simulink library "carma_platform"  (Simulink 8.2)
settings: Solver=ode1  StartTime=0.0  StopTime=Inf  FixedStep=0.001  RelTol=1e-3
PostLoadFcn:
  | , if any(exist('dsrtsu_mdlpostloadfcn', 'file') == [2, 3, 6]), try dsrtsu_mdlpostloadfcn('Execute', bdroot); catch fprintf('Error in PostLoadFcn (dsrtsu_mdlpostloadfcn) for model "%s":\n %s\n', bdroot, lasterr); end, end,
libraries: srx_platform x7, topr5_adapter x4, rtitttasklib x4, dsrc_handler x1, parse_utils x1, rtiethernetudplib x1
settings Model: DSRTSU_INTERNAL_RTI_VER=450  DSRTSU_INTERNAL_RTI_TYPE=rti1401  DSRTSU_INTERNAL_RTIFPGA=40  Creator=leidos  LastModifiedBy=rushk1

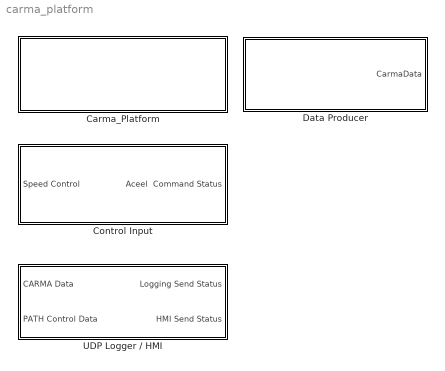
== system carma_platform ==
  "Carma_Platform " : Subsystem
  Control Input : Subsystem
  Data Producer : Subsystem  mask{Value=0.05}
      mask prompts: Value "Data Output Interval (s):"
      mask TypeOptions Value:
      | Triggered
      | Subsystem/Constant2/Value
  UDP Logger / HMI : Subsystem  mask{Value=0.05}
      mask prompts: Value "Output Interval (s):"
      mask TypeOptions Value: Subsystem/Constant2/Value

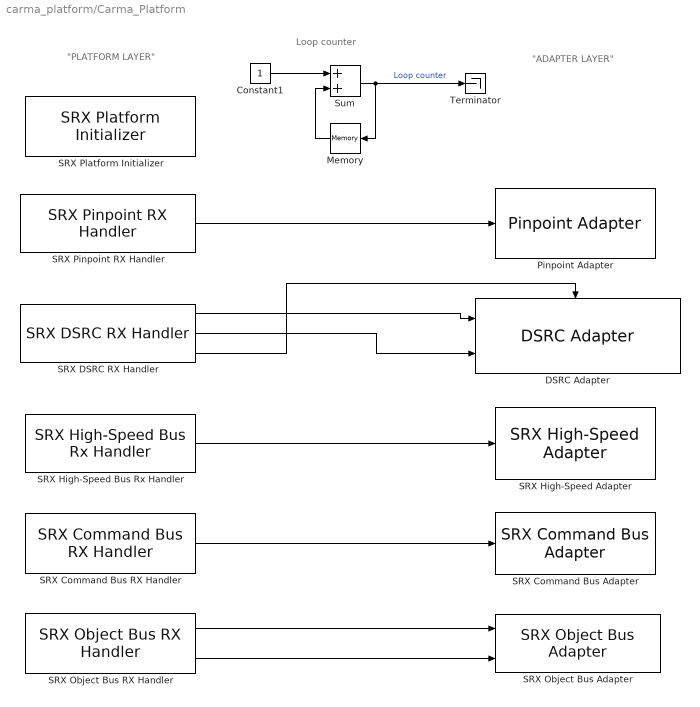
== system carma_platform/Carma_Platform  ==
  note: "ADAPTER LAYER"
  note: "PLATFORM LAYER"
  note: Loop counter
  Constant1 : Constant
  DSRC Adapter : dsrc_handler/DSRC Adapter
  Memory : Memory  InheritSampleTime=on
  Pinpoint Adapter : topr5_adapter/Pinpoint Adapter
  SRX Command Bus Adapter : topr5_adapter/SRX Command Bus Adapter
  SRX Command Bus RX Handler : srx_platform/SRX Command Bus RX Handler  SystemSampleTime=-1
  SRX DSRC RX Handler : srx_platform/SRX DSRC RX Handler
  SRX High-Speed Adapter : topr5_adapter/SRX High-Speed Adapter
  SRX High-Speed Bus Rx Handler : srx_platform/SRX High-Speed Bus Rx Handler  SystemSampleTime=-1
  SRX Object Bus Adapter : topr5_adapter/SRX Object Bus Adapter
  SRX Object Bus RX Handler : srx_platform/SRX Object Bus RX Handler
  SRX Pinpoint RX Handler : srx_platform/SRX Pinpoint RX Handler
  SRX Platform Initializer : srx_platform/SRX Platform Initializer  enable_can1=on  enable_can2=on  enable_can3=on  enable_can4=off
  Sum : Sum  SaturateOnIntegerOverflow=on  InputSameDT=on  OutDataTypeStr=Inherit: Same as first input
  Terminator : Terminator
  wires:
  SRX Pinpoint RX Handler/1 -> Pinpoint Adapter/1
  Sum/1 -> Terminator/1, Memory/1  "Loop counter"
  Memory/1 -> Sum/2
  Constant1/1 -> Sum/1
  SRX High-Speed Bus Rx Handler/1 -> SRX High-Speed Adapter/1
  SRX Command Bus RX Handler/1 -> SRX Command Bus Adapter/1
  SRX Object Bus RX Handler/1 -> SRX Object Bus Adapter/1
  SRX Object Bus RX Handler/2 -> SRX Object Bus Adapter/2
  SRX DSRC RX Handler/1 -> DSRC Adapter/1
  SRX DSRC RX Handler/2 -> DSRC Adapter/2
  SRX DSRC RX Handler/3 -> DSRC Adapter/Enable

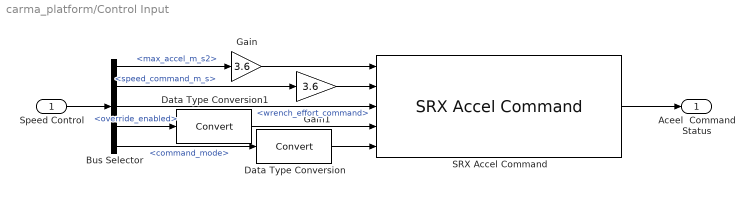
== system carma_platform/Control Input ==
  Speed Control : Inport  OutDataTypeStr=Bus: AccelCommandBus
  Bus Selector : BusSelector  OutputSignals=max_accel_m_s2,speed_command_m_s,wrench_effort_command,override_enabled,command_mode
  Data Type Conversion : DataTypeConversion
  Data Type Conversion1 : DataTypeConversion
  Gain : Gain  Gain=3.6
  Gain1 : Gain  Gain=3.6
  SRX Accel Command : srx_platform/SRX Accel Command
  Aceel  Command Status : Outport
  wires:
  SRX Accel Command/1 -> Aceel  Command Status/1
  Speed Control/1 -> Bus Selector/1
  Gain/1 -> SRX Accel Command/1
  Gain1/1 -> SRX Accel Command/2
  Bus Selector/1 -> Gain/1  "<max_accel_m_s2>"
  Bus Selector/2 -> Gain1/1  "<speed_command_m_s>"
  Bus Selector/3 -> SRX Accel Command/3  "<wrench_effort_command>"
  Bus Selector/4 -> Data Type Conversion1/1  "<override_enabled>"
  Bus Selector/5 -> Data Type Conversion/1  "<command_mode>"
  Data Type Conversion/1 -> SRX Accel Command/5
  Data Type Conversion1/1 -> SRX Accel Command/4

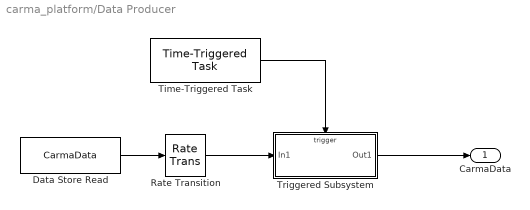
== system carma_platform/Data Producer ==
  Data Store Read : DataStoreRead  DataStoreName=CarmaData  SampleTime=0.01  DataStoreElements=CarmaData
  Rate Transition : RateTransition  Deterministic=off
  Time-Triggered Task : rtitttasklib/Time-Triggered Task  TimeTriggerId=data_prod  TLCFileName=rtitimetriggeredtask  DSProperties=struct('RTI',struct('Version',uint32(1),'BlockType',struct('isSLSource',uint8(1),'isSLSink',uint8(0),'isHWSource',uint8(0),'isHWSink',uint8(0),'isSetup',uint8(0),'isInline',uint8(1),'isNonInline',uint8(0),'isInterrupt',uint8(0),'isChannelwise',uint8(0)),'IOBoardType','RTITIMETRIGGER','UnitType','TIMETRIGGERED','Identifier','TASK','DialogType','SL','BlockSet','NONE','SlaveProcessor','NONE'))  RTIBlockInterface=struct('OutputPortsActive',1,'OutputPortsWidth',int32(1),'FunctionCall',uint32(0),'OutputPortsName',{{[' ']}},'InitLevel',3,'BlockDisplay',{{['Time-Triggered Task\nID: ''''data_prod'''''],'center'}},'IconTransparency','off','BlockName',struct('Token',{{['Time-Triggered Task']}}),'MaskDescription',['Specifies a time-triggered task. The task trigger times are set by the assigned Time-Trigger Set block.' char(10) '' char(10) 'This block can only be used together with the Time-Trigger Set block.'])  RTIBlockParameters=struct('TimeTriggerId',{{'data_prod','OFF',[]}},'TLCFileName',{{'rtitimetriggeredtask','OFF',[]}})  RTISFcnParameters=struct('TLCFileName','char')  RTIBlockParaDefault=struct('TimeTriggerId','TT_ID','TLCFileName','rtitimetriggeredtask')
  Triggered Subsystem : Subsystem  TreatAsAtomicUnit=on
  CarmaData : Outport
  wires:
  Rate Transition/1 -> Triggered Subsystem/1(In1)
  Data Store Read/1 -> Rate Transition/1
  Triggered Subsystem/1(Out1) -> CarmaData/1
  Time-Triggered Task/1 -> Triggered Subsystem/Trigger

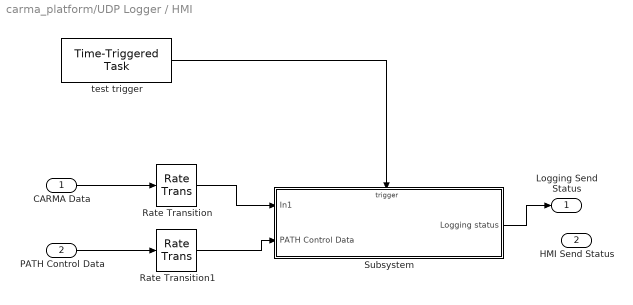
== system carma_platform/UDP Logger / HMI ==
  CARMA Data : Inport
  PATH Control Data : Inport  Port=2  PortDimensions=[74]
  Rate Transition : RateTransition  Deterministic=off
  Rate Transition1 : RateTransition  Deterministic=off
  Subsystem : Subsystem
  test trigger : rtitttasklib/Time-Triggered Task  TimeTriggerId=TT_ID  TLCFileName=rtitimetriggeredtask  DSProperties=struct('RTI',struct('Version',uint32(1),'BlockType',struct('isSLSource',uint8(1),'isSLSink',uint8(0),'isHWSource',uint8(0),'isHWSink',uint8(0),'isSetup',uint8(0),'isInline',uint8(1),'isNonInline',uint8(0),'isInterrupt',uint8(0),'isChannelwise',uint8(0)),'IOBoardType','RTITIMETRIGGER','UnitType','TIMETRIGGERED','Identifier','TASK','DialogType','SL','BlockSet','NONE','SlaveProcessor','NONE'))  RTIBlockInterface=struct('OutputPortsActive',1,'OutputPortsWidth',int32(1),'FunctionCall',uint32(0),'OutputPortsName',{{[' ']}},'InitLevel',3,'BlockDisplay',{{['Time-Triggered Task\nID: ''''TT_ID'''''],'center'}},'IconTransparency','off','BlockName',struct('Token',{{['Time-Triggered Task']}}),'MaskDescription',['Specifies a time-triggered task. The task trigger times are set by the assigned Time-Trigger Set block.' char(10) '' char(10) 'This block can only be used together with the Time-Trigger Set block.'])  RTIBlockParameters=struct('TimeTriggerId',{{'TT_ID','OFF',[]}},'TLCFileName',{{'rtitimetriggeredtask','OFF',[]}})  RTISFcnParameters=struct('TLCFileName','char')  RTIBlockParaDefault=struct('TimeTriggerId','TT_ID','TLCFileName','rtitimetriggeredtask')
  Logging Send Status : Outport
  HMI Send Status : Outport  Port=2
  wires:
  CARMA Data/1 -> Rate Transition/1
  Rate Transition/1 -> Subsystem/1(In1)
  test trigger/1 -> Subsystem/Trigger
  Rate Transition1/1 -> Subsystem/2(PATH Control Data)
  PATH Control Data/1 -> Rate Transition1/1
  Subsystem/1(Logging status) -> Logging Send Status/1
  ? -> HMI Send Status/1

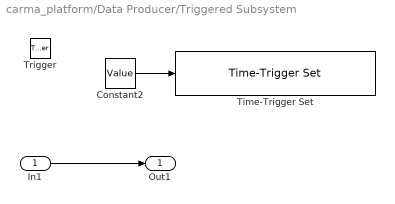
== system carma_platform/Data Producer/Triggered Subsystem ==
  In1 : Inport
  Trigger : TriggerPort  TriggerType=function-call
  Constant2 : Constant  Value=Value
  Time-Trigger Set : rtitttasklib/Time-Trigger Set  TimeTriggerId=data_prod  SampleTime=-1  RegisterAtSimulationStart=on  TLCFileName=rtitimetriggerset  DSProperties=struct('RTI',struct('Version',uint32(1),'BlockType',struct('isSLSource',uint8(1),'isSLSink',uint8(0),'isHWSource',uint8(0),'isHWSink',uint8(0),'isSetup',uint8(0),'isInline',uint8(1),'isNonInline',uint8(0),'isInterrupt',uint8(0),'isChannelwise',uint8(0)),'IOBoardType','RTITIMETRIGGER','UnitType','TIMETRIGGERED','Identifier','SET','DialogType','SL','BlockSet','NONE','SlaveProcessor','NONE'))  RTIBlockInterface=struct('InputPortsActive',1,'InputPortsWidth',{{'DYNAMICALLY_SIZED'}},'InputPortsDataType',{{'SS_DOUBLE'}},'InputPortsName',{{['Trigger delay']}},'InitLevel',3,'BlockDisplay',{{['Time-Trigger Set\nID: ''''data_prod'''''],'center'}},'IconTransparency','on','BlockName',struct('Token',{{['Time-Trigger Set']}}),'MaskDescription',['When this block is evaluated it sets the task trigger times for the assigned time-triggered task.' char(10) '' char(10) 'This block can only be used together with the Time-Triggered Task block.'],'SampleTime',{{-1}})  RTIBlockParameters=struct('TimeTriggerId',{{'data_prod','OFF',[]}},'SampleTime',{{-1,'OFF',[]}},'RegisterAtSimulationStart',{{logical(1),'OFF',[]}},'TLCFileName',{{'rtitimetriggerset','OFF',[]}})  RTISFcnParameters=struct('TimeTriggerId','char','SampleTime','double','TLCFileName','char','RegisterAtSimulationStart','double')  RTIBlockParaDefault=struct('TimeTriggerId','TT_ID','SampleTime',-1,'RegisterAtSimulationStart',0,'TLCFileName','rtitimetriggerset')
  Out1 : Outport
  wires:
  In1/1 -> Out1/1
  Constant2/1 -> Time-Trigger Set/1

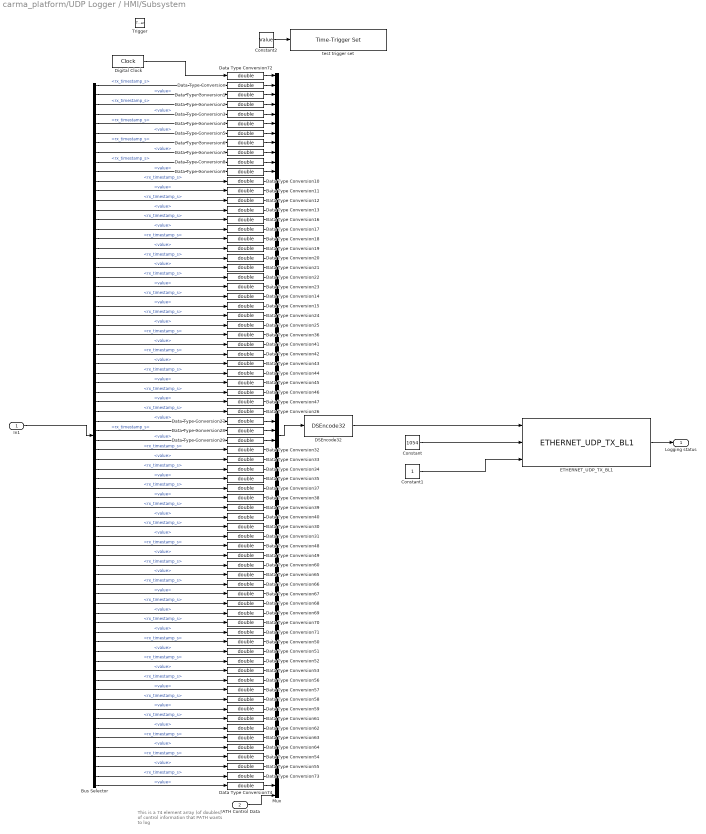
== system carma_platform/UDP Logger / HMI/Subsystem ==
  note: This is a 74 element array (of doubles)
      | of control information that
      | PATH wants to log
  In1 : Inport
  PATH Control Data : Inport  Port=2  PortDimensions=[74]
  Trigger : TriggerPort  TriggerType=function-call  PortDimensions=1
  Bus Selector : BusSelector  OutputSignals=radar_status.rx_timestamp_s,radar_status.value,acc_status.rx_timestamp_s,acc_status.value,path_ctrl_status.rx_timestamp_s,path_ctrl_status.value,throttle_ovr_flag.rx_timestamp_s,throttle_ovr_flag.value,acc_set_speed_m_s.rx_timestamp_s,acc_set_speed_m_s.value,accel_m_s2.rx_timestamp_s,accel_m_s2.value,speed_m_s.rx_timestamp_s,speed_m_s.value,steering_wheel_angle_deg.rx_timestamp_s,steering_wheel_angle_deg.value,brk_light_flag.rx_timestamp_s,brk_light_flag.value,brk_pedal_deflect_percent.rx_timestamp_s,brk_pedal_deflect_percent.value,throttle_pedal_deflect_percent.rx_timestamp_s,throttle_pedal_deflect_percent.value,global_utc_time_s.rx_timestamp_s,global_utc_time_s.value,global_lat_deg.rx_timestamp_s,global_lat_deg.value,global_long_deg.rx_timestamp_s,global_long_deg.value,global_alt_m.rx_timestamp_s,global_alt_m.value,global_roll_deg.rx_timestamp_s,global_roll_deg.value,global_pitch_deg.rx_timestamp_s,global_pitch_deg.value,global_yaw_deg.rx_timestamp_s,global_yaw_deg.value,local_north_m.rx_timestamp_s,local_north_m.value,local_east_m.rx_timestamp_s,local_east_m.value,local_down_m.rx_timestamp_s,local_down_m.value,local_roll_deg.rx_timestamp_s,local_roll_deg.value,local_pitch_deg.rx_timestamp_s,local_pitch_deg.value,local_yaw_deg.rx_timestamp_s,local_yaw_deg.value,horizontal_pos_accuracy_m.rx_timestamp_s,horizontal_pos_accuracy_m.value,vertical_pos_accuracy_m.rx_timestamp_s,vertical_pos_accuracy_m.value,velocity_fwd_m_s.rx_timestamp_s,velocity_fwd_m_s.value,velocity_right_m_s.rx_timestamp_s,velocity_right_m_s.value,velocity_down_m_s.rx_timestamp_s,velocity_down_m_s.value,velocity_accuracy_m_s.rx_timestamp_s,velocity_accuracy_m_s.value,accel_fwd_m_s2.rx_timestamp_s,accel_fwd_m_s2.value,accel_right_m_s2.rx_timestamp_s,accel_right_m_s2.value,accel_down_m_s2.rx_timestamp_s,accel_down_m_s2.value,dist_to_preceding_veh_m.rx_timestamp_s,dist_to_preceding_veh_m.value,rel_speed_to_preceding_veh_m_s.rx_timestamp_s,rel_speed_to_preceding_veh_m_s.value,desired_headway.rx_timestamp_s,desired_headway.value,requested_cacc_state.rx_timestamp_s,requested_cacc_state.value
  Constant : Constant  Value=1054  OutDataTypeStr=int32
  Constant1 : Constant  OutDataTypeStr=boolean
  Constant2 : Constant  Value=Value
  DSEncode32 : parse_utils/DSEncode32  byteordering=little endian (Intel)  offset=[ 0 ]  auto_offset=on  datatype=[9 9 3 9 3 9 3 9 3 9 8 9 8 9 8 9 8 9 3 9 8 9 8 9 9 9 9 9 9 9 9 9 8 9 8 9 8 9 9 9 9 9 9 9 8 9 8 9 8 9 8 9 8 9 8 9 8 9 8 9 8 9 8 9 8 9 8 9 8 9 8 9 6 9 3 9 9 9 9 9 9 9 9 9 9 9 9 9 9 9 9 9 9 9 9 9 9 9 9 9 9 9 9 9 9 9 9 9 9 9 9 9 9 9 9 9 9 9 9 9 9 9 9 9 9 9 9 9 9 9 9 9 9 9 9 9 9 9 9 9 9 9 9 9 9 9 9 9 9]  one_datatype=off  sampletime=-1
  Data Type Conversion{,1..74} (75 alike) : DataTypeConversion  OutDataTypeStr=double
  Digital Clock : DigitalClock  SampleTime=-1
  ETHERNET_UDP_TX_BL1 : rtiethernetudplib/ETHERNET_UDP_TX_BL1  InterfaceName=rti_ethernet_interface_name  BoardType=ETH Type 1  ModuleNo=1  ChannelNo=1  SocketNo=3  MaxMessageSize=1054  SendTimeout=0.0005  LocalSocket=192.168.88.21:5002  RemoteSocket=192.168.88.10:5002  DSProperties=struct('RTI',struct('Version',uint32(2),'BlockType',struct('isSLSource',uint8(1),'isSLSink',uint8(1),'isHWSource',uint8(1),'isHWSink',uint8(1),'isSetup',uint8(0),'isInline',uint8(1),'isNonInline',uint8(1),'isInterrupt',uint8(0),'isChannelwise',uint8(1)),'IOBoardType','DSETHERNETUDP','UnitType','ETHUDP','Identifier','TX','DialogType','SL','BlockSet','RTIETHERNETUDP','SlaveProcessor','NONE'))  RTIBlockInterface=struct('OutputPortsWidth',int32(1),'OutputPortsActive',1,'OutputPortsName',{{'Status'}},'OutputPortsDataType',{{'SS_UINT16'}},'InputPortsWidth',int32([1 1 1]),'InputPortsActive',[1 1 1],'InputPortsName',{{'Data',['Message Size'],'Enable'}},'InputPortsDataType',{{'SS_UINT32','SS_INT32','SS_BOOLEAN'}},'BlockDisplay',{{['Ethernet UDP Transmit\nBoard Type: ETH Type 1\nModule: 1\nSocket: 3\nMaximum Message Size: 1054'],'center'}},'IconTransparency','on','InitLevel',3,'BlockName',struct('Token',{{'ETHERNET_UDP_TX_BL1'}}),'MaskDescription',['To send messages via the Ethernet UDP interface.'])  RTIBlockParameters=struct('InterfaceName',{{'rti_ethernet_interface_name','OFF',[]}},'BoardType',{{1,'OFF',[]}},'ModuleNo',{{1,'OFF',[1 16]}},'ChannelNo',{{1,'OFF',[1 2]}},'SocketNo',{{3,'OFF',[1 4]}},'MaxMessageSize',{{1054,'ON',[1 1472]}},'SendTimeout',{{0.0005,'ON',[1e-05 2]}},'LocalSocket',{{'192.168.88.21:5002','OFF',[]}},'RemoteSocket',{{'192.168.88.10:5002','OFF',[]}})  RTISFcnParameters=struct('InterfaceName','char','BoardType','double','ModuleNo','double','ChannelNo','double','SocketNo','double','MaxMessageSize','double','SendTimeout','double','LocalSocket','char','RemoteSocket','char')  RTIBlockParaDefault=struct('InterfaceName','rti_ethernet_interface_name','BoardType',1,'ModuleNo',1,'ChannelNo',1,'SocketNo',1,'MaxMessageSize',625,'SendTimeout',0.0005,'LocalSocket','XXX.XXX.XXX.XXX:5000','RemoteSocket','XXX.XXX.XXX.XXX:5000')
  Mux : Mux  Inputs=76
  test trigger set : rtitttasklib/Time-Trigger Set  TimeTriggerId=TT_ID  SampleTime=-1  RegisterAtSimulationStart=on  TLCFileName=rtitimetriggerset  DSProperties=struct('RTI',struct('Version',uint32(1),'BlockType',struct('isSLSource',uint8(1),'isSLSink',uint8(0),'isHWSource',uint8(0),'isHWSink',uint8(0),'isSetup',uint8(0),'isInline',uint8(1),'isNonInline',uint8(0),'isInterrupt',uint8(0),'isChannelwise',uint8(0)),'IOBoardType','RTITIMETRIGGER','UnitType','TIMETRIGGERED','Identifier','SET','DialogType','SL','BlockSet','NONE','SlaveProcessor','NONE'))  RTIBlockInterface=struct('InputPortsActive',1,'InputPortsWidth',{{'DYNAMICALLY_SIZED'}},'InputPortsDataType',{{'SS_DOUBLE'}},'InputPortsName',{{['Trigger delay']}},'InitLevel',3,'BlockDisplay',{{['Time-Trigger Set\nID: ''''TT_ID'''''],'center'}},'IconTransparency','on','BlockName',struct('Token',{{['Time-Trigger Set']}}),'MaskDescription',['When this block is evaluated it sets the task trigger times for the assigned time-triggered task.' char(10) '' char(10) 'This block can only be used together with the Time-Triggered Task block.'],'SampleTime',{{-1}})  RTIBlockParameters=struct('TimeTriggerId',{{'TT_ID','OFF',[]}},'SampleTime',{{-1,'OFF',[]}},'RegisterAtSimulationStart',{{logical(1),'OFF',[]}},'TLCFileName',{{'rtitimetriggerset','OFF',[]}})  RTISFcnParameters=struct('TimeTriggerId','char','SampleTime','double','TLCFileName','char','RegisterAtSimulationStart','double')  RTIBlockParaDefault=struct('TimeTriggerId','TT_ID','SampleTime',-1,'RegisterAtSimulationStart',0,'TLCFileName','rtitimetriggerset')
  Logging status : Outport
  wires:
  DSEncode32/1 -> ETHERNET_UDP_TX_BL1/1
  Bus Selector/1 -> Data Type Conversion/1  "<rx_timestamp_s>"
  Bus Selector/43 -> Data Type Conversion37/1  "<rx_timestamp_s>"
  Bus Selector/6 -> Data Type Conversion5/1  "<value>"
  Bus Selector/3 -> Data Type Conversion2/1  "<rx_timestamp_s>"
  Bus Selector/2 -> Data Type Conversion1/1  "<value>"
  Bus Selector/39 -> Data Type Conversion32/1  "<rx_timestamp_s>"
  Bus Selector/23 -> Data Type Conversion14/1  "<rx_timestamp_s>"
  Bus Selector/69 -> Data Type Conversion63/1  "<rx_timestamp_s>"
  Bus Selector/24 -> Data Type Conversion15/1  "<value>"
  Bus Selector/61 -> Data Type Conversion52/1  "<rx_timestamp_s>"
  Bus Selector/7 -> Data Type Conversion6/1  "<rx_timestamp_s>"
  Bus Selector/20 -> Data Type Conversion21/1  "<value>"
  Bus Selector/10 -> Data Type Conversion9/1  "<value>"
  Bus Selector/71 -> Data Type Conversion54/1  "<rx_timestamp_s>"
  Bus Selector/12 -> Data Type Conversion11/1  "<value>"
  Bus Selector/49 -> Data Type Conversion48/1  "<rx_timestamp_s>"
  Bus Selector/44 -> Data Type Conversion38/1  "<value>"
  Bus Selector/48 -> Data Type Conversion31/1  "<value>"
  Bus Selector/4 -> Data Type Conversion3/1  "<value>"
  Bus Selector/8 -> Data Type Conversion7/1  "<value>"
  Bus Selector/33 -> Data Type Conversion46/1  "<rx_timestamp_s>"
  Bus Selector/29 -> Data Type Conversion42/1  "<rx_timestamp_s>"
  Bus Selector/56 -> Data Type Conversion69/1  "<value>"
  Bus Selector/53 -> Data Type Conversion66/1  "<rx_timestamp_s>"
  Bus Selector/11 -> Data Type Conversion10/1  "<rx_timestamp_s>"
  Bus Selector/36 -> Data Type Conversion27/1  "<value>"
  Bus Selector/51 -> Data Type Conversion60/1  "<rx_timestamp_s>"
  Bus Selector/18 -> Data Type Conversion19/1  "<value>"
  Bus Selector/26 -> Data Type Conversion25/1  "<value>"
  Bus Selector/67 -> Data Type Conversion61/1  "<rx_timestamp_s>"
  Bus Selector/72 -> Data Type Conversion55/1  "<value>"
  Bus Selector/59 -> Data Type Conversion50/1  "<rx_timestamp_s>"
  Bus Selector/64 -> Data Type Conversion57/1  "<value>"
  Bus Selector/21 -> Data Type Conversion22/1  "<rx_timestamp_s>"
  Bus Selector/46 -> Data Type Conversion40/1  "<value>"
  Bus Selector/34 -> Data Type Conversion47/1  "<value>"
  Bus Selector/13 -> Data Type Conversion12/1  "<rx_timestamp_s>"
  Bus Selector/57 -> Data Type Conversion70/1  "<rx_timestamp_s>"
  Bus Selector/54 -> Data Type Conversion67/1  "<value>"
  Bus Selector/5 -> Data Type Conversion4/1  "<rx_timestamp_s>"
  Bus Selector/30 -> Data Type Conversion43/1  "<value>"
  Bus Selector/35 -> Data Type Conversion26/1  "<rx_timestamp_s>"
  Bus Selector/38 -> Data Type Conversion29/1  "<value>"
  Bus Selector/14 -> Data Type Conversion13/1  "<value>"
  Bus Selector/28 -> Data Type Conversion41/1  "<value>"
  Bus Selector/52 -> Data Type Conversion65/1  "<value>"
  Bus Selector/17 -> Data Type Conversion18/1  "<rx_timestamp_s>"
  Bus Selector/15 -> Data Type Conversion16/1  "<rx_timestamp_s>"
  Bus Selector/45 -> Data Type Conversion39/1  "<rx_timestamp_s>"
  Bus Selector/19 -> Data Type Conversion20/1  "<rx_timestamp_s>"
  Bus Selector/42 -> Data Type Conversion35/1  "<value>"
  Bus Selector/50 -> Data Type Conversion49/1  "<value>"
  Bus Selector/55 -> Data Type Conversion68/1  "<rx_timestamp_s>"
  Bus Selector/65 -> Data Type Conversion58/1  "<rx_timestamp_s>"
  Bus Selector/66 -> Data Type Conversion59/1  "<value>"
  Bus Selector/62 -> Data Type Conversion53/1  "<value>"
  Bus Selector/58 -> Data Type Conversion71/1  "<value>"
  Bus Selector/27 -> Data Type Conversion36/1  "<rx_timestamp_s>"
  Bus Selector/40 -> Data Type Conversion33/1  "<value>"
  Bus Selector/22 -> Data Type Conversion23/1  "<value>"
  Bus Selector/32 -> Data Type Conversion45/1  "<value>"
  Bus Selector/9 -> Data Type Conversion8/1  "<rx_timestamp_s>"
  Bus Selector/60 -> Data Type Conversion51/1  "<value>"
  Bus Selector/47 -> Data Type Conversion30/1  "<rx_timestamp_s>"
  Bus Selector/63 -> Data Type Conversion56/1  "<rx_timestamp_s>"
  Bus Selector/37 -> Data Type Conversion28/1  "<rx_timestamp_s>"
  Bus Selector/16 -> Data Type Conversion17/1  "<value>"
  Bus Selector/25 -> Data Type Conversion24/1  "<rx_timestamp_s>"
  Bus Selector/31 -> Data Type Conversion44/1  "<rx_timestamp_s>"
  Bus Selector/41 -> Data Type Conversion34/1  "<rx_timestamp_s>"
  Mux/1 -> DSEncode32/1
  Constant/1 -> ETHERNET_UDP_TX_BL1/2
  Constant1/1 -> ETHERNET_UDP_TX_BL1/3
  ETHERNET_UDP_TX_BL1/1 -> Logging status/1
  In1/1 -> Bus Selector/1
  Constant2/1 -> test trigger set/1
  Digital Clock/1 -> Data Type Conversion72/1
  Data Type Conversion39/1 -> Mux/46
  Data Type Conversion/1 -> Mux/2
  Data Type Conversion1/1 -> Mux/3
  Data Type Conversion10/1 -> Mux/12
  Data Type Conversion11/1 -> Mux/13
  Data Type Conversion12/1 -> Mux/14
  Data Type Conversion13/1 -> Mux/15
  Data Type Conversion14/1 -> Mux/24
  Data Type Conversion15/1 -> Mux/25
  Data Type Conversion16/1 -> Mux/16
  Data Type Conversion17/1 -> Mux/17
  Data Type Conversion18/1 -> Mux/18
  Data Type Conversion19/1 -> Mux/19
  Data Type Conversion2/1 -> Mux/4
  Data Type Conversion20/1 -> Mux/20
  Data Type Conversion21/1 -> Mux/21
  Data Type Conversion22/1 -> Mux/22
  Data Type Conversion23/1 -> Mux/23
  Data Type Conversion24/1 -> Mux/26
  Data Type Conversion25/1 -> Mux/27
  Data Type Conversion26/1 -> Mux/36
  Data Type Conversion27/1 -> Mux/37
  Data Type Conversion28/1 -> Mux/38
  Data Type Conversion29/1 -> Mux/39
  Data Type Conversion3/1 -> Mux/5
  Data Type Conversion30/1 -> Mux/48
  Data Type Conversion31/1 -> Mux/49
  Data Type Conversion32/1 -> Mux/40
  Data Type Conversion33/1 -> Mux/41
  Data Type Conversion34/1 -> Mux/42
  Data Type Conversion35/1 -> Mux/43
  Data Type Conversion36/1 -> Mux/28
  Data Type Conversion37/1 -> Mux/44
  Data Type Conversion38/1 -> Mux/45
  Data Type Conversion4/1 -> Mux/6
  Data Type Conversion40/1 -> Mux/47
  Data Type Conversion41/1 -> Mux/29
  Data Type Conversion42/1 -> Mux/30
  Data Type Conversion43/1 -> Mux/31
  Data Type Conversion44/1 -> Mux/32
  Data Type Conversion45/1 -> Mux/33
  Data Type Conversion46/1 -> Mux/34
  Data Type Conversion47/1 -> Mux/35
  Data Type Conversion48/1 -> Mux/50
  Data Type Conversion49/1 -> Mux/51
  Data Type Conversion5/1 -> Mux/7
  Data Type Conversion50/1 -> Mux/60
  Data Type Conversion51/1 -> Mux/61
  Data Type Conversion52/1 -> Mux/62
  Data Type Conversion53/1 -> Mux/63
  Data Type Conversion54/1 -> Mux/72
  Data Type Conversion55/1 -> Mux/73
  Data Type Conversion56/1 -> Mux/64
  Data Type Conversion57/1 -> Mux/65
  Data Type Conversion58/1 -> Mux/66
  Data Type Conversion59/1 -> Mux/67
  Data Type Conversion6/1 -> Mux/8
  Data Type Conversion60/1 -> Mux/52
  Data Type Conversion61/1 -> Mux/68
  Data Type Conversion62/1 -> Mux/69
  Data Type Conversion63/1 -> Mux/70
  Data Type Conversion64/1 -> Mux/71
  Data Type Conversion65/1 -> Mux/53
  Data Type Conversion66/1 -> Mux/54
  Data Type Conversion67/1 -> Mux/55
  Data Type Conversion68/1 -> Mux/56
  Data Type Conversion69/1 -> Mux/57
  Data Type Conversion7/1 -> Mux/9
  Data Type Conversion70/1 -> Mux/58
  Data Type Conversion71/1 -> Mux/59
  Data Type Conversion8/1 -> Mux/10
  Data Type Conversion9/1 -> Mux/11
  Data Type Conversion72/1 -> Mux/1
  PATH Control Data/1 -> Mux/76
  Bus Selector/73 -> Data Type Conversion73/1  "<rx_timestamp_s>"
  Data Type Conversion73/1 -> Mux/74
  Data Type Conversion74/1 -> Mux/75
  Bus Selector/74 -> Data Type Conversion74/1  "<value>"
  Bus Selector/68 -> Data Type Conversion62/1  "<value>"
  Bus Selector/70 -> Data Type Conversion64/1  "<value>"
